simulink model "SimuOrbital"  (R2020b)
settings: Solver=VariableStepAuto  StartTime=0.0  StopTime=20000  RelTol=1e-3
model workspace (MAT data in the model file):
  Ang0 = [0; 0; 0]
  VelAng0 = [0; 0; 0]
  altura = 3.5
  delta = 0.05
  mu = 0.01
  r = 2.25
  radio = 2.25
libraries: sharedutil x11, aerolibutil x4, simulink_extras x3, sharedtransform x3, aerolibbdyn x2, vrlib x1, simulink x1
settings Model: Creator=Sergio  LastModifiedBy=Sergio
settings SolverCC: ZeroCrossAlgorithm=Adaptive

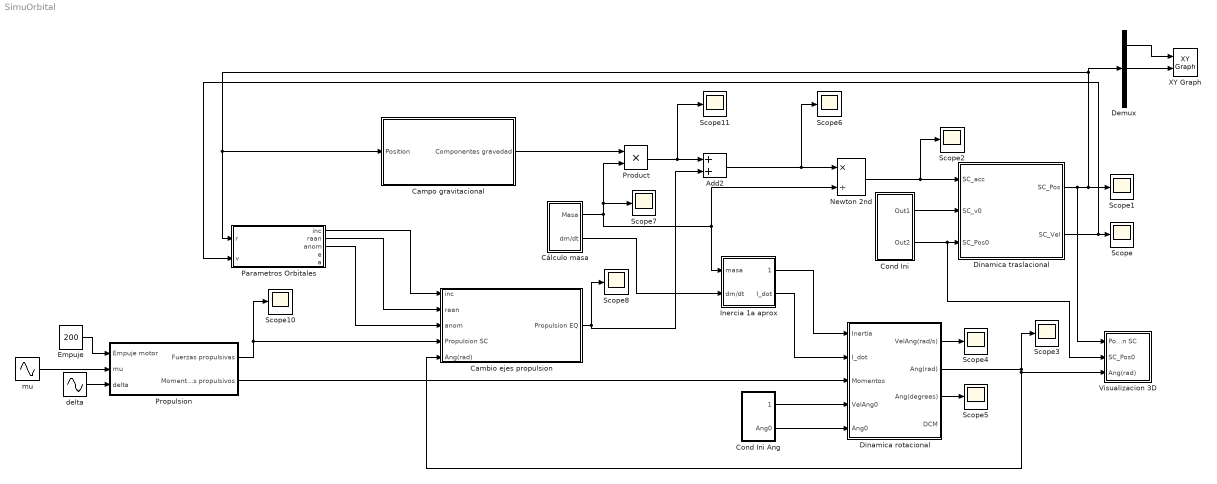
== system SimuOrbital ==
  Add2 : Sum
  Cambio ejes propulsion : Subsystem
  Campo gravitacional : Subsystem
  Cond Ini : Subsystem  mask{v0=[-1636,0,0], Pos0=[0,1837100,0]}
  Cond Ini Ang : Subsystem  mask{VelAng0=[0,0,0], Ang0=[0,0,0]}
  Cálculo masa : Subsystem
  Demux : Demux  Outputs=3
  Dinamica rotacional : Subsystem
  Dinamica traslacional : Subsystem
  Empuje : Constant  Value=200
  Inercia 1a aprox : Subsystem
  Newton 2nd : Product  Inputs=*/
  Parametros Orbitales : Subsystem
  Product : Product
  Propulsion : Subsystem
  Scope{,1..8,10..11} (11 alike) : Scope
  Visualizacion 3D : Subsystem
  XY Graph : simulink/Sinks/XY Graph  xmin=-2500000  xmax=2500000  ymin=-2500000  ymax=2500000  st=-1
  delta : Sin  Amplitude=0.01  Frequency=0.001  SampleTime=0
  mu : Sin  Amplitude=0.05  Frequency=0.001  SampleTime=0
  wires:
  Cond Ini/1(Out1) -> Dinamica traslacional/2(SC_v0)
  Cond Ini/2(Out2) -> Visualizacion 3D/2(SC_Pos0), Dinamica traslacional/3(SC_Pos0)
  Newton 2nd/1 -> Scope2/1, Dinamica traslacional/1(SC_acc)
  Dinamica traslacional/2(SC_Vel) -> Parametros Orbitales/2(v), Scope/1
  Inercia 1a aprox/1(Inertia) -> Dinamica rotacional/1(Inertia)
  Dinamica rotacional/1(VelAng(rad/s)) -> Scope4/1
  Cond Ini Ang/1(VelAng0) -> Dinamica rotacional/4(VelAng0)
  Cond Ini Ang/2(Ang0) -> Dinamica rotacional/5(Ang0)
  Dinamica rotacional/3(Ang(degrees)) -> Scope5/1
  Empuje/1 -> Propulsion/1(Empuje motor)
  Campo gravitacional/1(Componentes gravedad) -> Product/1
  Add2/1 -> Scope6/1, Newton 2nd/1
  Dinamica traslacional/1(SC_Pos) -> Visualizacion 3D/1(Posicion SC), Demux/1, Campo gravitacional/1(Position), Parametros Orbitales/1(r), Scope1/1
  Demux/1 -> XY Graph/1
  Demux/2 -> XY Graph/2
  Cambio ejes propulsion/1(Propulsion EQ) -> Add2/2, Scope8/1
  Parametros Orbitales/2(raan) -> Cambio ejes propulsion/2(raan)
  Parametros Orbitales/1(inc) -> Cambio ejes propulsion/1(inc)
  Parametros Orbitales/3(anom) -> Cambio ejes propulsion/3(anom)
  Dinamica rotacional/2(Ang(rad)) -> Cambio ejes propulsion/5(Ang(rad)), Visualizacion 3D/3(Ang(rad)), Scope3/1
  Propulsion/1(Fuerzas propulsivas) -> Scope10/1, Cambio ejes propulsion/4(Propulsion SC)
  Inercia 1a aprox/2(I_dot) -> Dinamica rotacional/2(I_dot)
  Cálculo masa/1(Masa) -> Inercia 1a aprox/1(masa), Newton 2nd/2, Scope7/1, Product/2
  Cálculo masa/2(dm/dt) -> Inercia 1a aprox/2(dm/dt)
  Product/1 -> Scope11/1, Add2/1
  Propulsion/2(Momentos propulsivos) -> Dinamica rotacional/3(Momentos)
  mu/1 -> Propulsion/2(mu)
  delta/1 -> Propulsion/3(delta)

== system SimuOrbital/Cambio ejes propulsion ==
  inc : Inport
  raan : Inport  Port=2
  anom : Inport  Port=3
  Propulsion SC : Inport  Port=4
  Ang(rad) : Inport  Port=5
  MATLAB Function : MATLAB Function  Commented=on  TreatAsAtomicUnit=on
  MatrixMultiply : Product  Inputs=3  Multiplication=Matrix(*)
  Product2 : Product  Multiplication=Matrix(*)
  Subsystem : Subsystem
  Subsystem1 : Subsystem
  Subsystem2 : Subsystem
  Propulsion EQ : Outport
  wires:
  inc/1 -> Subsystem/1(inc)
  raan/1 -> Subsystem/2(raan)
  anom/1 -> Subsystem1/1(anom)
  Ang(rad)/1 -> Subsystem2/1(ang)
  Subsystem/1(Ropeq) -> MatrixMultiply/1
  Subsystem1/1(Rloop) -> MatrixMultiply/2
  MatrixMultiply/1 -> Product2/1
  Product2/1 -> Propulsion EQ/1
  Subsystem2/1(Ralo) -> MatrixMultiply/3
  Propulsion SC/1 -> Product2/2

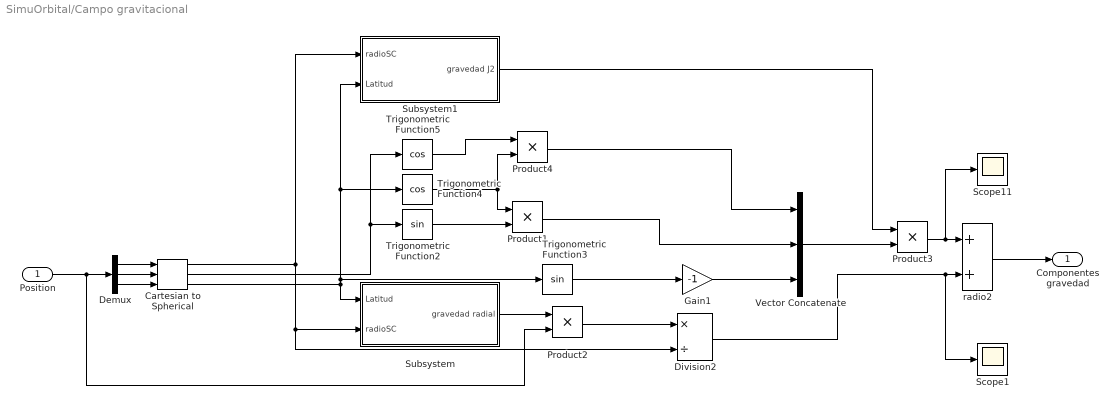
== system SimuOrbital/Campo gravitacional ==
  Position : Inport
  Cartesian to Spherical : simulink_extras/Transformations/Cartesian to Spherical
      settings: SourceProductBaseCode=SL
  Demux : Demux  Outputs=3
  Division2 : Product  Inputs=*/
  Gain1 : Gain  Gain=-1
  Product{1..4} (4 alike) : Product
  Scope1 : Scope
  Scope11 : Scope
  Subsystem : Subsystem
  Subsystem1 : Subsystem
  Trigonometric Function2 : Trigonometry
  Trigonometric Function3 : Trigonometry
  Trigonometric Function4 : Trigonometry  Operator=cos
  Trigonometric Function5 : Trigonometry  Operator=cos
  Vector Concatenate : Concatenate  NumInputs=3
  radio2 : Sum
  Componentes gravedad : Outport
  wires:
  Cartesian to Spherical/3 -> Subsystem/1(Latitud), Subsystem1/2(Latitud), Trigonometric Function4/1, Trigonometric Function3/1
  Position/1 -> Product2/2, Demux/1
  Cartesian to Spherical/1 -> Subsystem/2(radioSC), Division2/2, Subsystem1/1(radioSC)
  Product2/1 -> Division2/1
  Demux/2 -> Cartesian to Spherical/2
  Demux/1 -> Cartesian to Spherical/1
  Demux/3 -> Cartesian to Spherical/3
  Subsystem/1(gravedad radial) -> Product2/1
  Division2/1 -> Scope1/1, radio2/2
  radio2/1 -> Componentes gravedad/1
  Product3/1 -> Scope11/1, radio2/1
  Subsystem1/1(gravedad J2) -> Product3/1
  Trigonometric Function4/1 -> Product4/2, Product1/1
  Trigonometric Function2/1 -> Product1/2
  Cartesian to Spherical/2 -> Trigonometric Function5/1, Trigonometric Function2/1
  Trigonometric Function5/1 -> Product4/1
  Product4/1 -> Vector Concatenate/1
  Product1/1 -> Vector Concatenate/2
  Gain1/1 -> Vector Concatenate/3
  Trigonometric Function3/1 -> Gain1/1
  Vector Concatenate/1 -> Product3/2

== system SimuOrbital/Cond Ini ==
  SC_Pos0 : Constant  Value=Pos0  VectorParams1D=off
  SC_v0 : Constant  Value=v0  VectorParams1D=off
  Out1 : Outport
  Out2 : Outport  Port=2
  wires:
  SC_Pos0/1 -> Out2/1
  SC_v0/1 -> Out1/1

== system SimuOrbital/Cond Ini Ang ==
  CIAng : Constant  Value=Ang0  VectorParams1D=off
  CIVelAng : Constant  Value=VelAng0  VectorParams1D=off
  VelAng0 : Outport
  Ang0 : Outport  Port=2
  wires:
  CIVelAng/1 -> VelAng0/1
  CIAng/1 -> Ang0/1

== system SimuOrbital/Cálculo masa ==
  Add : Sum  Inputs=+-
  Constant : Constant
  Integrator : Integrator
  Masa inicial : Constant  Value=5000
  Masa seca : Constant  Value=2530
  Product : Product
  Switch : Switch  Criteria=u2 > Threshold  Threshold=2530
  dm/dt (kg/s) : Constant  Value=0
  Masa : Outport
  dm/dt : Outport  Port=2
  wires:
  dm/dt (kg/s)/1 -> Product/2, dm/dt/1
  Masa seca/1 -> Switch/3
  Switch/1 -> Masa/1
  Constant/1 -> Integrator/1
  Integrator/1 -> Product/1
  Product/1 -> Add/2
  Masa inicial/1 -> Add/1
  Add/1 -> Switch/2, Switch/1

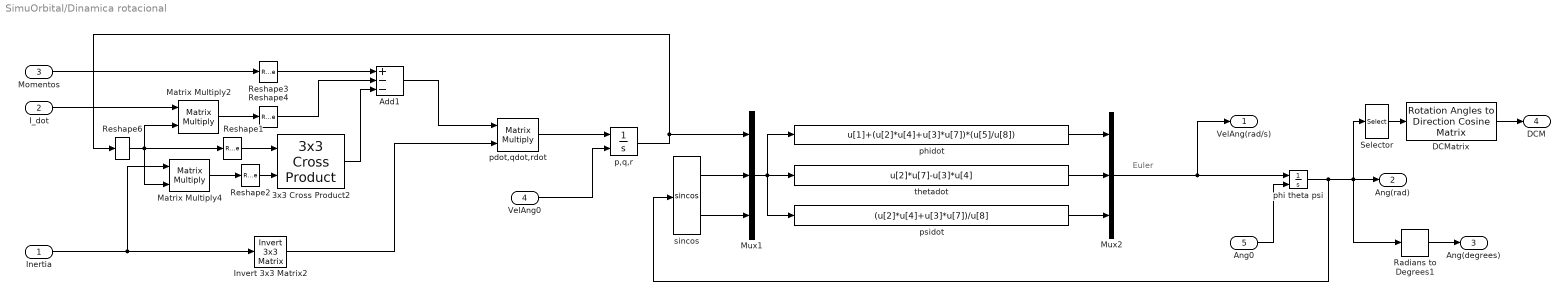
== system SimuOrbital/Dinamica rotacional ==
  note: Euler
  Inertia : Inport
  I_dot : Inport  Port=2
  Momentos : Inport  Port=3
  VelAng0 : Inport  Port=4
  Ang0 : Inport  Port=5
  3x3 Cross Product2 : sharedutil/3x3 Cross Product  aMode=aMode
      settings: SourceProductBaseCode=AE,PW,MT,UV,VE,VP
  Add1 : Sum  Inputs=+--
  DCMatrix : sharedtransform/Rotation Angles to Direction Cosine Matrix  rotationOrder=ZYX  aMode=aMode
      settings: SourceProductBaseCode=AE,PW,MT,UV,VE,VP
  Invert 3x3 Matrix2 : aerolibutil/Invert  3x3 Matrix
  Matrix Multiply2 : Product  Multiplication=Matrix(*)
  Matrix Multiply4 : Product  Multiplication=Matrix(*)
  Mux1 : Mux  Inputs=[3 3 3]
  Mux2 : Mux  Inputs=3
  Radians to Degrees1 : simulink_extras/Transformations/Radians to Degrees
  Reshape{1..4} (4 alike) : Reshape  OutputDimensionality=Row vector (2-D)
  Reshape6 : Reshape  OutputDimensionality=Column vector (2-D)
  Selector : Selector  InputPortWidth=3  IndexOptions=Index vector (dialog)  Indices=[3 2 1]  OutputSizes=1
  p,q,r : Integrator  InitialConditionSource=external
  pdot,qdot,rdot : Product  Multiplication=Matrix(*)
  phi theta psi : Integrator  InitialConditionSource=external  WrapState=on
  phidot : Fcn  Expr=u[1]+(u[2]*u[4]+u[3]*u[7])*(u[5]/u[8])
  psidot : Fcn  Expr=(u[2]*u[4]+u[3]*u[7])/u[8]
  sincos : Trigonometry  Operator=sincos
  thetadot : Fcn  Expr=u[2]*u[7]-u[3]*u[4]
  VelAng(rad/s) : Outport
  Ang(rad) : Outport  Port=2
  Ang(degrees) : Outport  Port=3
  DCM : Outport  Port=4
  wires:
  Invert 3x3 Matrix2/1 -> pdot,qdot,rdot/2
  Inertia/1 -> Matrix Multiply4/1, Invert 3x3 Matrix2/1
  Add1/1 -> pdot,qdot,rdot/1
  pdot,qdot,rdot/1 -> p,q,r/1
  I_dot/1 -> Matrix Multiply2/1
  3x3 Cross Product2/1 -> Add1/3
  Mux1/1 -> thetadot/1, phidot/1, psidot/1
  sincos/2 -> Mux1/3
  sincos/1 -> Mux1/2
  thetadot/1 -> Mux2/2
  phidot/1 -> Mux2/1
  psidot/1 -> Mux2/3
  Radians to Degrees1/1 -> Ang(degrees)/1
  Ang0/1 -> phi theta psi/2
  Mux2/1 -> phi theta psi/1, VelAng(rad/s)/1
  p,q,r/1 -> Reshape6/1, Mux1/1
  Reshape1/1 -> 3x3 Cross Product2/1
  Matrix Multiply4/1 -> Reshape2/1
  Reshape2/1 -> 3x3 Cross Product2/2
  Reshape3/1 -> Add1/1
  Momentos/1 -> Reshape3/1
  Matrix Multiply2/1 -> Reshape4/1
  Reshape4/1 -> Add1/2
  VelAng0/1 -> p,q,r/2
  Reshape6/1 -> Matrix Multiply2/2, Matrix Multiply4/2, Reshape1/1
  phi theta psi/1 -> Radians to Degrees1/1, Selector/1, Ang(rad)/1, sincos/1
  Selector/1 -> DCMatrix/1
  DCMatrix/1 -> DCM/1

== system SimuOrbital/Dinamica traslacional ==
  SC_acc : Inport
  SC_v0 : Inport  Port=2
  SC_Pos0 : Inport  Port=3
  Add : Sum
  Add1 : Sum
  Integrator : Integrator
  Integrator1 : Integrator
  SC_Pos : Outport
  SC_Vel : Outport  Port=2
  wires:
  Add/1 -> SC_Vel/1, Integrator1/1
  Add1/1 -> SC_Pos/1
  SC_Pos0/1 -> Add1/2
  SC_acc/1 -> Integrator/1
  SC_v0/1 -> Add/2
  Integrator/1 -> Add/1
  Integrator1/1 -> Add1/1

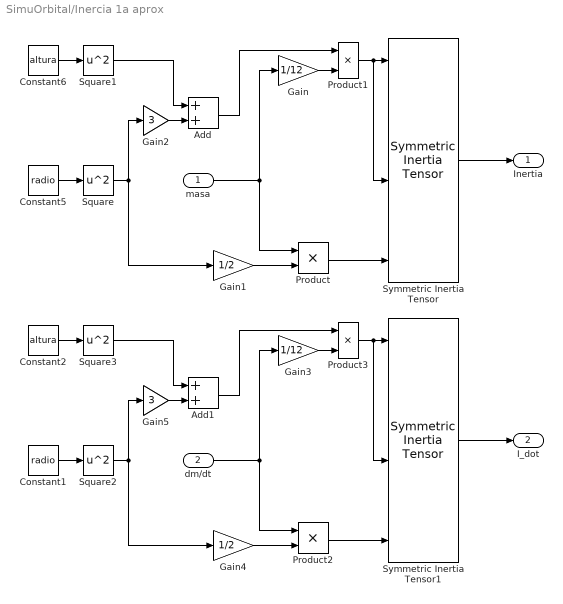
== system SimuOrbital/Inercia 1a aprox ==
  masa : Inport
  dm/dt : Inport  Port=2
  Add : Sum
  Add1 : Sum
  Constant1 : Constant  Value=radio
  Constant2 : Constant  Value=altura
  Constant5 : Constant  Value=radio
  Constant6 : Constant  Value=altura
  Gain : Gain  Gain=1/12
  Gain1 : Gain  Gain=1/2
  Gain2 : Gain  Gain=3
  Gain3 : Gain  Gain=1/12
  Gain4 : Gain  Gain=1/2
  Gain5 : Gain  Gain=3
  Product{,1..3} (4 alike) : Product
  Square{,1..3} (4 alike) : Math  Operator=square  SaturateOnIntegerOverflow=on
  Symmetric Inertia Tensor : aerolibbdyn/Symmetric Inertia Tensor
      settings: SourceProductBaseCode=AE
  Symmetric Inertia Tensor1 : aerolibbdyn/Symmetric Inertia Tensor
      settings: SourceProductBaseCode=AE
  Inertia : Outport
  I_dot : Outport  Port=2
  wires:
  Gain2/1 -> Add/2
  Square1/1 -> Add/1
  Product/1 -> Symmetric Inertia Tensor/6
  masa/1 -> Gain/1, Product/1
  Gain/1 -> Product1/2
  Symmetric Inertia Tensor/1 -> Inertia/1
  Square/1 -> Gain2/1, Gain1/1
  Add/1 -> Product1/1
  Product1/1 -> Symmetric Inertia Tensor/4, Symmetric Inertia Tensor/1
  Gain1/1 -> Product/2
  Constant5/1 -> Square/1
  Constant6/1 -> Square1/1
  Constant1/1 -> Square2/1
  Square2/1 -> Gain5/1, Gain4/1
  Constant2/1 -> Square3/1
  Square3/1 -> Add1/1
  Product3/1 -> Symmetric Inertia Tensor1/4, Symmetric Inertia Tensor1/1
  Gain5/1 -> Add1/2
  Gain3/1 -> Product3/2
  Gain4/1 -> Product2/2
  Product2/1 -> Symmetric Inertia Tensor1/6
  Add1/1 -> Product3/1
  dm/dt/1 -> Gain3/1, Product2/1
  Symmetric Inertia Tensor1/1 -> I_dot/1

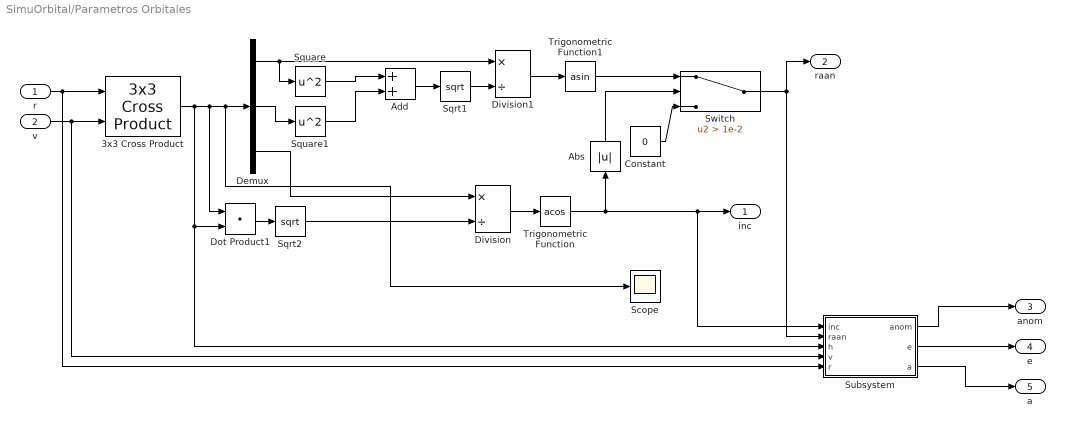
== system SimuOrbital/Parametros Orbitales ==
  r : Inport
  v : Inport  Port=2
  3x3 Cross Product : sharedutil/3x3 Cross Product  aMode=aMode
      settings: SourceProductBaseCode=AE,PW,MT,UV,VE,VP
  Abs : Abs
  Add : Sum
  Constant : Constant  Value=0
  Demux : Demux  Outputs=3
  Division : Product  Inputs=*/
  Division1 : Product  Inputs=*/
  Dot Product1 : DotProduct  InputSameDT=on  OutDataTypeStr=Inherit: Inherit via internal rule
  Scope : Scope
  Sqrt1 : Sqrt  SaturateOnIntegerOverflow=on
  Sqrt2 : Sqrt  SaturateOnIntegerOverflow=on
  Square : Math  Operator=square  SaturateOnIntegerOverflow=on
  Square1 : Math  Operator=square  SaturateOnIntegerOverflow=on
  Subsystem : Subsystem
  Switch : Switch  Criteria=u2 > Threshold  Threshold=1e-2
  Trigonometric Function : Trigonometry  Operator=acos
  Trigonometric Function1 : Trigonometry  Operator=asin
  inc : Outport
  raan : Outport  Port=2
  anom : Outport  Port=3
  e : Outport  Port=4
  a : Outport  Port=5
  wires:
  r/1 -> Subsystem/5(r), 3x3 Cross Product/1
  Trigonometric Function/1 -> Abs/1, Subsystem/1(inc), inc/1
  Division/1 -> Trigonometric Function/1
  Demux/3 -> Division/1
  Sqrt2/1 -> Division/2
  Switch/1 -> Subsystem/2(raan), raan/1
  Dot Product1/1 -> Sqrt2/1
  v/1 -> Subsystem/4(v), 3x3 Cross Product/2
  Constant/1 -> Switch/3
  Trigonometric Function1/1 -> Switch/1
  Abs/1 -> Switch/2
  Division1/1 -> Trigonometric Function1/1
  Demux/1 -> Square/1, Division1/1
  Sqrt1/1 -> Division1/2
  Add/1 -> Sqrt1/1
  Demux/2 -> Square1/1
  Square1/1 -> Add/2
  Square/1 -> Add/1
  Subsystem/2(e) -> e/1
  Subsystem/1(anom) -> anom/1
  Subsystem/3(a) -> a/1
  3x3 Cross Product/1 -> Subsystem/3(h), Dot Product1/2, Dot Product1/1, Scope/1, Demux/1

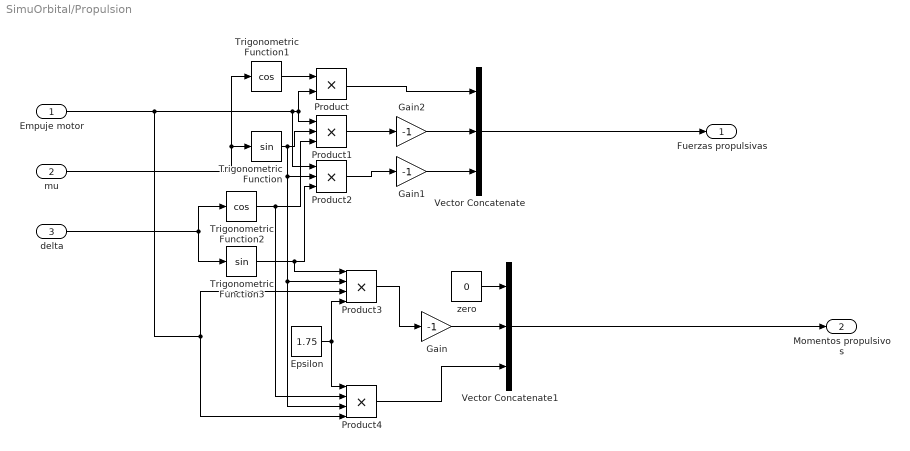
== system SimuOrbital/Propulsion ==
  Empuje motor : Inport
  mu : Inport  Port=2
  delta : Inport  Port=3
  Epsilon : Constant  Value=1.75
  Gain : Gain  Gain=-1
  Gain1 : Gain  Gain=-1
  Gain2 : Gain  Gain=-1
  Product : Product
  Product1 : Product  Inputs=3
  Product2 : Product  Inputs=3
  Product3 : Product  Inputs=4
  Product4 : Product  Inputs=4
  Trigonometric Function : Trigonometry
  Trigonometric Function1 : Trigonometry  Operator=cos
  Trigonometric Function2 : Trigonometry  Operator=cos
  Trigonometric Function3 : Trigonometry
  Vector Concatenate : Concatenate  NumInputs=3
  Vector Concatenate1 : Concatenate  NumInputs=3
  zero : Constant  Value=0
  Fuerzas propulsivas : Outport
  Momentos propulsivos : Outport  Port=2
  wires:
  Product4/1 -> Vector Concatenate1/3
  zero/1 -> Vector Concatenate1/1
  Trigonometric Function1/1 -> Product/1
  Vector Concatenate1/1 -> Momentos propulsivos/1
  delta/1 -> Trigonometric Function2/1, Trigonometric Function3/1
  Trigonometric Function/1 -> Product4/3, Product3/2, Product2/2, Product1/2
  Empuje motor/1 -> Product4/4, Product3/3, Product2/1, Product/2, Product1/1
  Trigonometric Function3/1 -> Product3/1, Product2/3
  mu/1 -> Trigonometric Function/1, Trigonometric Function1/1
  Trigonometric Function2/1 -> Product4/2, Product1/3
  Epsilon/1 -> Product3/4, Product4/1
  Product/1 -> Vector Concatenate/1
  Vector Concatenate/1 -> Fuerzas propulsivas/1
  Gain1/1 -> Vector Concatenate/3
  Gain2/1 -> Vector Concatenate/2
  Product1/1 -> Gain2/1
  Product2/1 -> Gain1/1
  Gain/1 -> Vector Concatenate1/2
  Product3/1 -> Gain/1

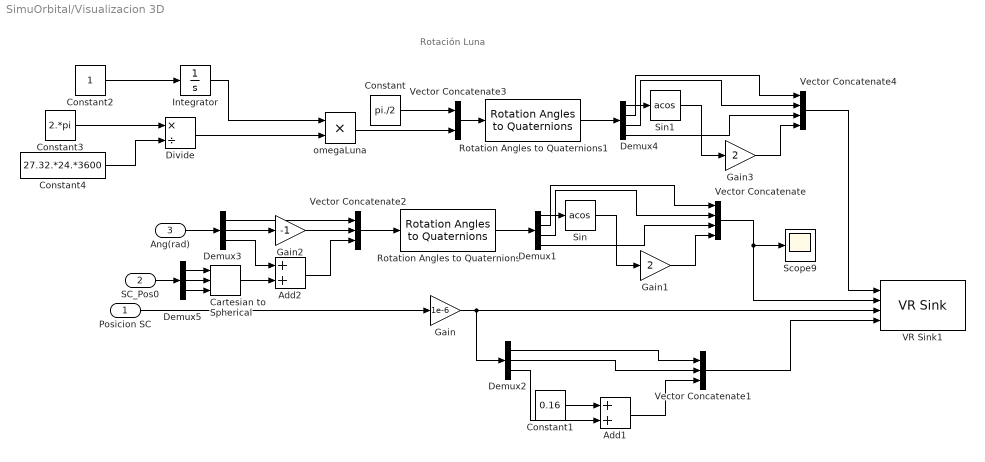
== system SimuOrbital/Visualizacion 3D ==
  note: Rotación Luna
  Posicion SC : Inport
  SC_Pos0 : Inport  Port=2
  Ang(rad) : Inport  Port=3
  Add1 : Sum
  Add2 : Sum
  Cartesian to Spherical : simulink_extras/Transformations/Cartesian to Spherical
      settings: SourceProductBaseCode=SL
  Constant : Constant  Value=pi./2
  Constant1 : Constant  Value=0.16
  Constant2 : Constant
  Constant3 : Constant  Value=2.*pi
  Constant4 : Constant  Value=27.32.*24.*3600
  Demux1 : Demux
  Demux2 : Demux  Outputs=3
  Demux3 : Demux  Outputs=3
  Demux4 : Demux
  Demux5 : Demux  Outputs=3
  Divide : Product  Inputs=*/
  Gain : Gain  Gain=1e-6
  Gain1 : Gain  Gain=2
  Gain2 : Gain  Gain=-1
  Gain3 : Gain  Gain=2
  Integrator : Integrator
  Rotation Angles to Quaternions : sharedtransform/Rotation Angles to Quaternions  rotationOrder=ZYZ  aMode=aMode
      settings: SourceProductBaseCode=AE,PW,MT,UV,VE,VP
  Rotation Angles to Quaternions1 : sharedtransform/Rotation Angles to Quaternions  rotationOrder=XYZ  aMode=aMode
      settings: SourceProductBaseCode=AE,PW,MT,UV,VE,VP
  Scope9 : Scope
  Sin : Trigonometry  Operator=acos
  Sin1 : Trigonometry  Operator=acos
  VR Sink1 : vrlib/VR Sink  InstantiateOnLoad=on  SampleTime=0.1  ViewEnable=on  RemoteChange=off  RemoteView=off  FieldsWritten=MOON.rotation.4.1.1.double#SC.rotation.4.1.1.double#SC.translation.3.1.1.double#Orbita_0001.position.3.1.1.double  WorldFileName=orbita.x3d  AutoView=off  VideoDimensions=[]  AllowVariableSize=off
  Vector Concatenate : Concatenate  NumInputs=4
  Vector Concatenate1 : Concatenate  NumInputs=3
  Vector Concatenate2 : Concatenate  NumInputs=3
  Vector Concatenate3 : Concatenate  NumInputs=3
  Vector Concatenate4 : Concatenate  NumInputs=4
  omegaLuna : Product
  wires:
  Constant1/1 -> Add1/1
  Demux2/2 -> Vector Concatenate1/2
  Demux1/3 -> Vector Concatenate/2
  Vector Concatenate1/1 -> VR Sink1/4
  Demux1/1 -> Sin/1
  Demux2/3 -> Add1/2
  Add1/1 -> Vector Concatenate1/3
  Gain/1 -> VR Sink1/3, Demux2/1
  Gain1/1 -> Vector Concatenate/4
  Demux1/4 -> Vector Concatenate/3
  Vector Concatenate/1 -> VR Sink1/2, Scope9/1
  Sin/1 -> Gain1/1
  Demux2/1 -> Vector Concatenate1/1
  Rotation Angles to Quaternions/1 -> Demux1/1
  Demux1/2 -> Vector Concatenate/1
  Posicion SC/1 -> Gain/1
  Ang(rad)/1 -> Demux3/1
  Vector Concatenate2/1 -> Rotation Angles to Quaternions/1
  Demux3/1 -> Vector Concatenate2/1
  Gain2/1 -> Vector Concatenate2/2
  Demux3/2 -> Gain2/1
  Vector Concatenate3/1 -> Rotation Angles to Quaternions1/1
  Rotation Angles to Quaternions1/1 -> Demux4/1
  Sin1/1 -> Gain3/1
  Demux4/2 -> Vector Concatenate4/1
  Gain3/1 -> Vector Concatenate4/4
  Demux4/3 -> Vector Concatenate4/2
  Demux4/4 -> Vector Concatenate4/3
  Demux4/1 -> Sin1/1
  Constant/1 -> Vector Concatenate3/1
  omegaLuna/1 -> Vector Concatenate3/3
  Constant2/1 -> Integrator/1
  Integrator/1 -> omegaLuna/1
  Divide/1 -> omegaLuna/2
  Constant3/1 -> Divide/1
  Constant4/1 -> Divide/2
  Vector Concatenate4/1 -> VR Sink1/1
  Demux3/3 -> Add2/1
  Add2/1 -> Vector Concatenate2/3
  Demux5/1 -> Cartesian to Spherical/1
  Demux5/2 -> Cartesian to Spherical/2
  Demux5/3 -> Cartesian to Spherical/3
  Cartesian to Spherical/2 -> Add2/2
  SC_Pos0/1 -> Demux5/1

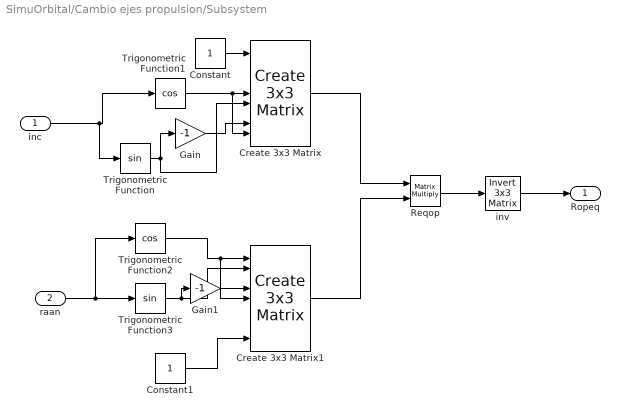
== system SimuOrbital/Cambio ejes propulsion/Subsystem ==
  inc : Inport
  raan : Inport  Port=2
  Constant : Constant
  Constant1 : Constant
  Create 3x3 Matrix : sharedutil/Create 3x3 Matrix  aMode=aMode
      settings: SourceProductBaseCode=AE,PW,MT,UV,VE,VP
  Create 3x3 Matrix1 : sharedutil/Create 3x3 Matrix  aMode=aMode
      settings: SourceProductBaseCode=AE,PW,MT,UV,VE,VP
  Gain : Gain  Gain=-1
  Gain1 : Gain  Gain=-1
  Reqop : Product  Multiplication=Matrix(*)
  Trigonometric Function : Trigonometry
  Trigonometric Function1 : Trigonometry  Operator=cos
  Trigonometric Function2 : Trigonometry  Operator=cos
  Trigonometric Function3 : Trigonometry
  inv : aerolibutil/Invert  3x3 Matrix
  Ropeq : Outport
  wires:
  Constant/1 -> Create 3x3 Matrix/1
  Trigonometric Function1/1 -> Create 3x3 Matrix/9, Create 3x3 Matrix/5
  inc/1 -> Trigonometric Function/1, Trigonometric Function1/1
  Trigonometric Function/1 -> Gain/1, Create 3x3 Matrix/6
  Constant1/1 -> Create 3x3 Matrix1/9
  Trigonometric Function2/1 -> Create 3x3 Matrix1/5, Create 3x3 Matrix1/1
  Trigonometric Function3/1 -> Gain1/1, Create 3x3 Matrix1/2
  Gain1/1 -> Create 3x3 Matrix1/4
  raan/1 -> Trigonometric Function2/1, Trigonometric Function3/1
  Create 3x3 Matrix/1 -> Reqop/1
  Create 3x3 Matrix1/1 -> Reqop/2
  Reqop/1 -> inv/1
  inv/1 -> Ropeq/1
  Gain/1 -> Create 3x3 Matrix/8

== system SimuOrbital/Cambio ejes propulsion/Subsystem1 ==
  anom : Inport
  Constant1 : Constant
  Constant2 : Constant
  Constant3 : Constant
  Create 3x3 Matrix1 : sharedutil/Create 3x3 Matrix  aMode=aMode
      settings: SourceProductBaseCode=AE,PW,MT,UV,VE,VP
  Create 3x3 Matrix2 : sharedutil/Create 3x3 Matrix  aMode=aMode
      settings: SourceProductBaseCode=AE,PW,MT,UV,VE,VP
  Create 3x3 Matrix3 : sharedutil/Create 3x3 Matrix  aMode=aMode
      settings: SourceProductBaseCode=AE,PW,MT,UV,VE,VP
  Gain1 : Gain  Gain=-1
  Gain2 : Gain  Gain=-1
  Gain3 : Gain  Gain=-1
  Roplo : Product  Inputs=3  Multiplication=Matrix(*)
  Trigonometric Function2 : Trigonometry  Operator=cos
  Trigonometric Function3 : Trigonometry
  inv : aerolibutil/Invert  3x3 Matrix
  Rloop : Outport
  wires:
  anom/1 -> Trigonometric Function2/1, Trigonometric Function3/1
  Constant3/1 -> Create 3x3 Matrix3/9
  Gain3/1 -> Create 3x3 Matrix3/4
  Trigonometric Function3/1 -> Gain3/1, Create 3x3 Matrix3/2
  Trigonometric Function2/1 -> Create 3x3 Matrix3/5, Create 3x3 Matrix3/1
  Create 3x3 Matrix2/1 -> Roplo/2
  Create 3x3 Matrix3/1 -> Roplo/3
  Create 3x3 Matrix1/1 -> Roplo/1
  inv/1 -> Rloop/1
  Roplo/1 -> inv/1
  Constant2/1 -> Create 3x3 Matrix2/8, Gain2/1, Create 3x3 Matrix2/1
  Gain2/1 -> Create 3x3 Matrix2/6
  Gain1/1 -> Create 3x3 Matrix1/7
  Constant1/1 -> Create 3x3 Matrix1/3, Create 3x3 Matrix1/5, Gain1/1

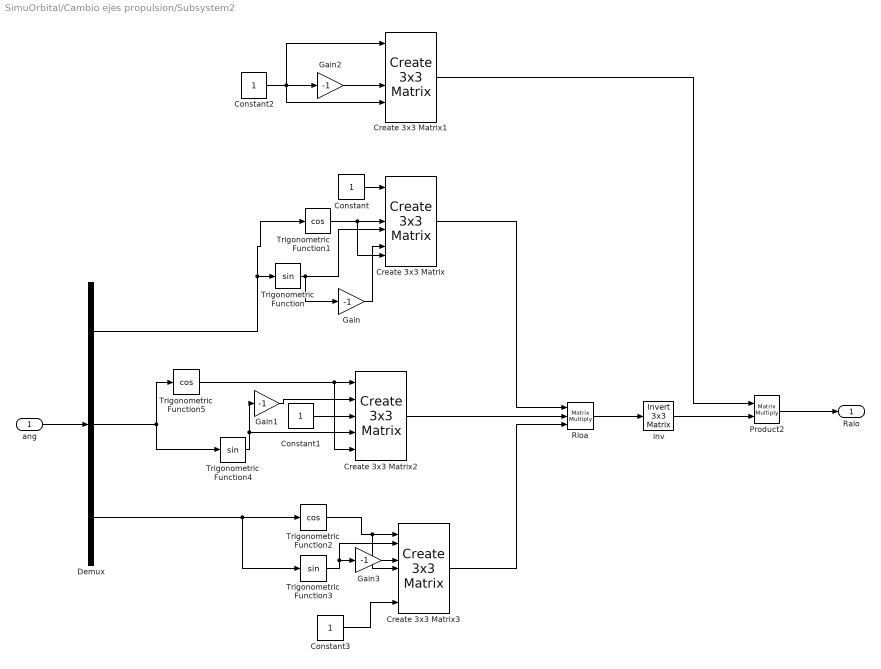
== system SimuOrbital/Cambio ejes propulsion/Subsystem2 ==
  ang : Inport
  Constant{,1..3} (4 alike) : Constant
  Create 3x3 Matrix{,1..3} (4 alike) : sharedutil/Create 3x3 Matrix  aMode=aMode
      settings: SourceProductBaseCode=AE,PW,MT,UV,VE,VP
  Demux : Demux  Outputs=3
  Gain{,1..3} (4 alike) : Gain  Gain=-1
  Product2 : Product  Multiplication=Matrix(*)
  Rloa : Product  Inputs=3  Multiplication=Matrix(*)
  Trigonometric Function : Trigonometry
  Trigonometric Function1 : Trigonometry  Operator=cos
  Trigonometric Function2 : Trigonometry  Operator=cos
  Trigonometric Function3 : Trigonometry
  Trigonometric Function4 : Trigonometry
  Trigonometric Function5 : Trigonometry  Operator=cos
  inv : aerolibutil/Invert  3x3 Matrix
  Ralo : Outport
  wires:
  Create 3x3 Matrix2/1 -> Rloa/2
  Constant3/1 -> Create 3x3 Matrix3/9
  Gain3/1 -> Create 3x3 Matrix3/4
  Trigonometric Function3/1 -> Gain3/1, Create 3x3 Matrix3/2
  Create 3x3 Matrix3/1 -> Rloa/3
  Trigonometric Function2/1 -> Create 3x3 Matrix3/5, Create 3x3 Matrix3/1
  ang/1 -> Demux/1
  Trigonometric Function/1 -> Create 3x3 Matrix/6, Gain/1
  Constant/1 -> Create 3x3 Matrix/1
  Trigonometric Function1/1 -> Create 3x3 Matrix/9, Create 3x3 Matrix/5
  Demux/1 -> Trigonometric Function1/1, Trigonometric Function/1
  Create 3x3 Matrix/1 -> Rloa/1
  Demux/3 -> Trigonometric Function3/1, Trigonometric Function2/1
  Constant1/1 -> Create 3x3 Matrix2/5
  Demux/2 -> Trigonometric Function4/1, Trigonometric Function5/1
  Trigonometric Function4/1 -> Create 3x3 Matrix2/7, Gain1/1
  Gain1/1 -> Create 3x3 Matrix2/3
  Trigonometric Function5/1 -> Create 3x3 Matrix2/9, Create 3x3 Matrix2/1
  Gain/1 -> Create 3x3 Matrix/8
  Constant2/1 -> Create 3x3 Matrix1/8, Create 3x3 Matrix1/1, Gain2/1
  Create 3x3 Matrix1/1 -> Product2/1
  Product2/1 -> Ralo/1
  inv/1 -> Product2/2
  Rloa/1 -> inv/1
  Gain2/1 -> Create 3x3 Matrix1/6

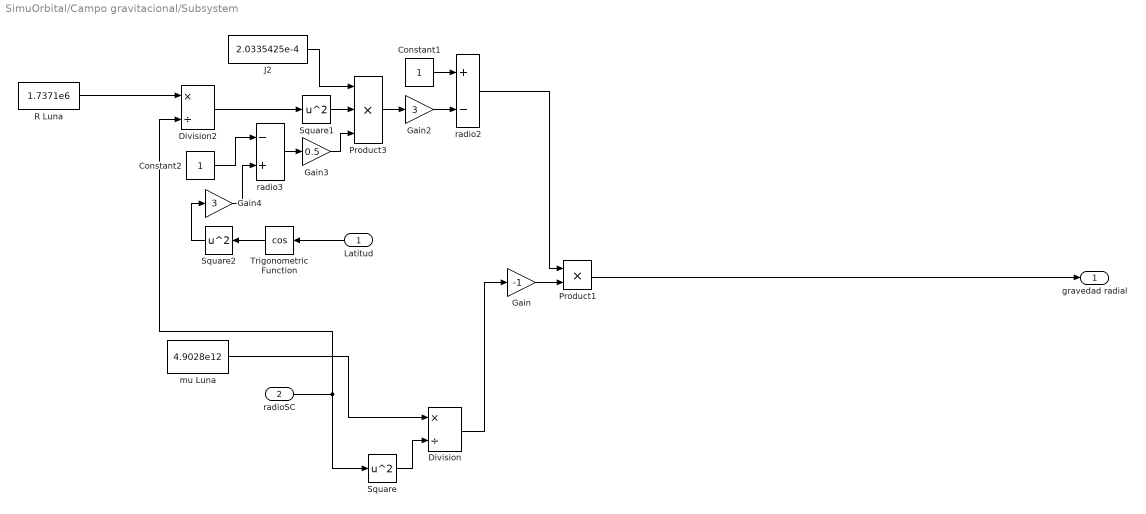
== system SimuOrbital/Campo gravitacional/Subsystem ==
  Latitud : Inport
  radioSC : Inport  Port=2
  Constant1 : Constant
  Constant2 : Constant
  Division : Product  Inputs=*/
  Division2 : Product  Inputs=*/
  Gain : Gain  Gain=-1
  Gain2 : Gain  Gain=3
  Gain3 : Gain  Gain=0.5
  Gain4 : Gain  Gain=3
  J2 : Constant  Value=2.0335425e-4
  Product1 : Product
  Product3 : Product  Inputs=3
  R Luna : Constant  Value=1.7371e6
  Square : Math  Operator=square  SaturateOnIntegerOverflow=on
  Square1 : Math  Operator=square  SaturateOnIntegerOverflow=on
  Square2 : Math  Operator=square  SaturateOnIntegerOverflow=on
  Trigonometric Function : Trigonometry  Operator=cos
  mu Luna : Constant  Value=4.9028e12
  radio2 : Sum  Inputs=+-
  radio3 : Sum  Inputs=-+
  gravedad radial : Outport
  wires:
  radio2/1 -> Product1/1
  R Luna/1 -> Division2/1
  mu Luna/1 -> Division/1
  Gain3/1 -> Product3/3
  radioSC/1 -> Square/1, Division2/2
  J2/1 -> Product3/1
  Division2/1 -> Square1/1
  Square1/1 -> Product3/2
  Division/1 -> Gain/1
  Constant1/1 -> radio2/1
  Latitud/1 -> Trigonometric Function/1
  Product3/1 -> Gain2/1
  Gain2/1 -> radio2/2
  Trigonometric Function/1 -> Square2/1
  Gain/1 -> Product1/2
  radio3/1 -> Gain3/1
  Square/1 -> Division/2
  Constant2/1 -> radio3/1
  Square2/1 -> Gain4/1
  Gain4/1 -> radio3/2
  Product1/1 -> gravedad radial/1

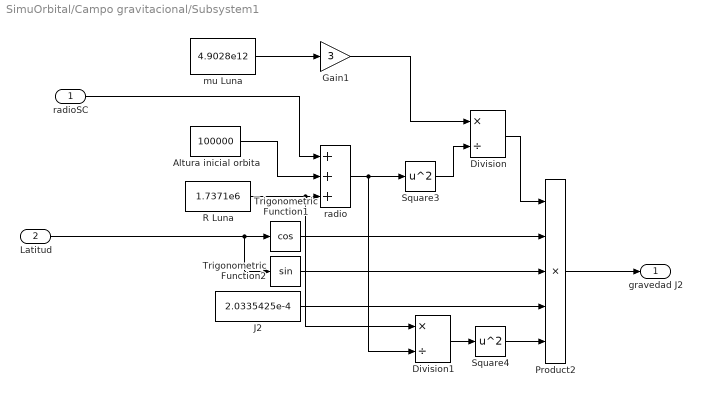
== system SimuOrbital/Campo gravitacional/Subsystem1 ==
  radioSC : Inport
  Latitud : Inport  Port=2
  Altura inicial orbita : Constant  Value=100000
  Division : Product  Inputs=*/
  Division1 : Product  Inputs=*/
  Gain1 : Gain  Gain=3
  J2 : Constant  Value=2.0335425e-4
  Product2 : Product  Inputs=5
  R Luna : Constant  Value=1.7371e6
  Square3 : Math  Operator=square  SaturateOnIntegerOverflow=on
  Square4 : Math  Operator=square  SaturateOnIntegerOverflow=on
  Trigonometric Function1 : Trigonometry  Operator=cos
  Trigonometric Function2 : Trigonometry
  mu Luna : Constant  Value=4.9028e12
  radio : Sum  Inputs=+++
  gravedad J2 : Outport
  wires:
  mu Luna/1 -> Gain1/1
  radioSC/1 -> radio/1
  R Luna/1 -> Division1/1, radio/3
  radio/1 -> Division1/2, Square3/1
  Division/1 -> Product2/1
  Square3/1 -> Division/2
  Altura inicial orbita/1 -> radio/2
  Gain1/1 -> Division/1
  Latitud/1 -> Trigonometric Function2/1, Trigonometric Function1/1
  Trigonometric Function1/1 -> Product2/2
  Trigonometric Function2/1 -> Product2/3
  J2/1 -> Product2/4
  Square4/1 -> Product2/5
  Division1/1 -> Square4/1
  Product2/1 -> gravedad J2/1

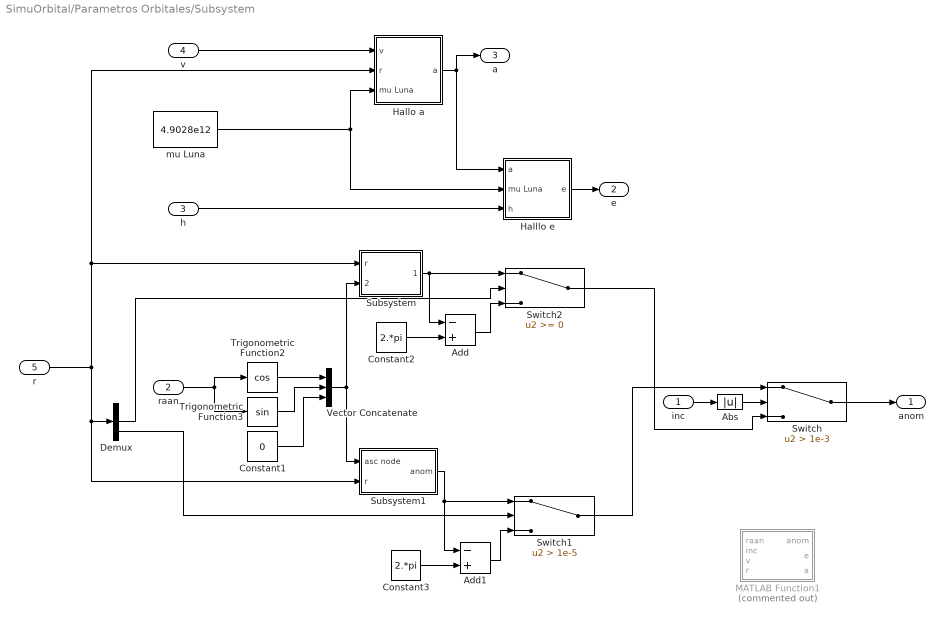
== system SimuOrbital/Parametros Orbitales/Subsystem ==
  inc : Inport
  raan : Inport  Port=2
  h : Inport  Port=3
  v : Inport  Port=4
  r : Inport  Port=5
  Abs : Abs
  Add : Sum  Inputs=-+
  Add1 : Sum  Inputs=-+
  Constant1 : Constant  Value=0
  Constant2 : Constant  Value=2.*pi
  Constant3 : Constant  Value=2.*pi
  Demux : Demux  Outputs=3
  Halllo e : Subsystem
  Hallo a : Subsystem
  MATLAB Function1 : MATLAB Function  Commented=on  TreatAsAtomicUnit=on
  Subsystem : Subsystem
  Subsystem1 : Subsystem
  Switch : Switch  Criteria=u2 > Threshold  Threshold=1e-3
  Switch1 : Switch  Criteria=u2 > Threshold  Threshold=1e-5
  Switch2 : Switch
  Trigonometric Function2 : Trigonometry  Operator=cos
  Trigonometric Function3 : Trigonometry
  Vector Concatenate : Concatenate  NumInputs=3
  mu Luna : Constant  Value=4.9028e12
  anom : Outport
  e : Outport  Port=2
  a : Outport  Port=3
  wires:
  Hallo a/1(a) -> Halllo e/1(a), a/1
  v/1 -> Hallo a/1(v)
  r/1 -> Hallo a/2(r), Subsystem/1(r), Subsystem1/2(r), Demux/1
  mu Luna/1 -> Hallo a/3(mu Luna), Halllo e/2(mu Luna)
  h/1 -> Halllo e/3(h)
  Halllo e/1(e) -> e/1
  inc/1 -> Abs/1
  Abs/1 -> Switch/2
  raan/1 -> Trigonometric Function3/1, Trigonometric Function2/1
  Trigonometric Function2/1 -> Vector Concatenate/1
  Trigonometric Function3/1 -> Vector Concatenate/2
  Constant1/1 -> Vector Concatenate/3
  Demux/3 -> Switch1/2
  Demux/2 -> Switch2/2
  Subsystem/1(anom) -> Add/1, Switch2/1
  Vector Concatenate/1 -> Subsystem1/1(asc node), Subsystem/2(asc node)
  Add/1 -> Switch2/3
  Constant2/1 -> Add/2
  Subsystem1/1(anom) -> Switch1/1, Add1/1
  Constant3/1 -> Add1/2
  Add1/1 -> Switch1/3
  Switch/1 -> anom/1
  Switch1/1 -> Switch/1
  Switch2/1 -> Switch/3

== system SimuOrbital/Parametros Orbitales/Subsystem/Halllo e ==
  a : Inport
  mu Luna : Inport  Port=2
  h : Inport  Port=3
  Constant1 : Constant
  Division4 : Product  Inputs=*/
  Dot Product3 : DotProduct  InputSameDT=on  OutDataTypeStr=Inherit: Inherit via internal rule
  Product1 : Product
  Sqrt1 : Sqrt  SaturateOnIntegerOverflow=on
  radio3 : Sum  Inputs=+-
  e : Outport
  wires:
  Dot Product3/1 -> Division4/1
  Constant1/1 -> radio3/1
  Product1/1 -> Division4/2
  Division4/1 -> radio3/2
  h/1 -> Dot Product3/2, Dot Product3/1
  radio3/1 -> Sqrt1/1
  Sqrt1/1 -> e/1
  mu Luna/1 -> Product1/2
  a/1 -> Product1/1

== system SimuOrbital/Parametros Orbitales/Subsystem/Hallo a ==
  v : Inport
  r : Inport  Port=2
  mu Luna : Inport  Port=3
  Division1 : Product  Inputs=*/
  Division3 : Product  Inputs=*/
  Dot Product1 : DotProduct  InputSameDT=on  OutDataTypeStr=Inherit: Inherit via internal rule
  Dot Product2 : DotProduct  InputSameDT=on  OutDataTypeStr=Inherit: Inherit via internal rule
  Gain2 : Gain  Gain=2
  Sqrt : Sqrt  SaturateOnIntegerOverflow=on
  radio2 : Sum  Inputs=+-
  a : Outport
  wires:
  v/1 -> Dot Product1/2, Dot Product1/1
  Dot Product1/1 -> radio2/2
  mu Luna/1 -> Gain2/1, Division1/1
  radio2/1 -> Division1/2
  r/1 -> Dot Product2/2, Dot Product2/1
  Gain2/1 -> Division3/1
  Division3/1 -> radio2/1
  Division1/1 -> a/1
  Dot Product2/1 -> Sqrt/1
  Sqrt/1 -> Division3/2

== system SimuOrbital/Parametros Orbitales/Subsystem/Subsystem ==
  r : Inport
  asc node : Inport  Port=2
  Divide : Product  Inputs=*/
  Dot Product : DotProduct  InputSameDT=on  OutDataTypeStr=Inherit: Inherit via internal rule
  Dot Product1 : DotProduct  InputSameDT=on  OutDataTypeStr=Inherit: Inherit via internal rule
  Sqrt : Sqrt  SaturateOnIntegerOverflow=on
  Trigonometric Function : Trigonometry  Operator=acos
  anom : Outport
  wires:
  Trigonometric Function/1 -> anom/1
  Divide/1 -> Trigonometric Function/1
  Sqrt/1 -> Divide/2
  Dot Product/1 -> Sqrt/1
  r/1 -> Dot Product/2, Dot Product1/2, Dot Product/1
  asc node/1 -> Dot Product1/1
  Dot Product1/1 -> Divide/1

== system SimuOrbital/Parametros Orbitales/Subsystem/Subsystem1 ==
  asc node : Inport
  r : Inport  Port=2
  Divide : Product  Inputs=*/
  Dot Product : DotProduct  InputSameDT=on  OutDataTypeStr=Inherit: Inherit via internal rule
  Dot Product1 : DotProduct  InputSameDT=on  OutDataTypeStr=Inherit: Inherit via internal rule
  Sqrt : Sqrt  SaturateOnIntegerOverflow=on
  Trigonometric Function : Trigonometry  Operator=acos
  anom : Outport
  wires:
  r/1 -> Dot Product1/2, Dot Product/1, Dot Product/2
  Divide/1 -> Trigonometric Function/1
  Dot Product/1 -> Sqrt/1
  Trigonometric Function/1 -> anom/1
  Sqrt/1 -> Divide/2
  asc node/1 -> Dot Product1/1
  Dot Product1/1 -> Divide/1

== matlab function SimuOrbital/Parametros Orbitales/Subsystem/MATLAB Function1 ==
  data: raan input; inc input; v input; r input; anom output; e output; a output
function [anom,e,a] = fcn(raan,inc,v,r)
    
    rnorm = abs(norm(r));
    vnorm = abs(norm(v));

    h = cross(r,v);
    hnorm = abs(norm(h));
    
    muLuna = 4.9028e12;
    
    p = (hnorm.^2)./muLuna;
    
    a = muLuna./(2.*muLuna./rnorm - vnorm.^2);
    
    e = sqrt(1 - p./a);
    
    ascnode = [cos(raan),sin(raan),0]; %Ascending node
    
    if abs(inc) > 1e-8
        if r(3) > 1e-5
            anom = acos((ascnode*r')./rnorm);
        else
            anom = 2.*pi - acos((ascnode*r')./rnorm);
        end    
    else
        if r(2) >= 0
            anom = acos((ascnode*r')./rnorm);
        else
            anom = 2.*pi - acos((ascnode*r')./rnorm);
        end 
    end
    

    
end

== matlab function SimuOrbital/Cambio ejes propulsion/MATLAB Function ==
  data: inc input; raan input; anom input; fsc input; feq output; ang input
function feq = fcn(inc,raan,anom,fsc,ang)

Reqop = [1,0,0;0,cos(inc),sin(inc);0,-sin(inc),cos(inc)]*[cos(raan),sin(raan),0;-sin(raan),cos(raan),0;0,0,1];
Ropeq = inv(Reqop);

Roplo = [1,0,0;0,0,-1;0,1,0]*[0,1,0;-1,0,0;0,0,1]*[cos(anom),sin(anom),0;-sin(anom),cos(anom),0;0,0,1];
Rloop = inv(Roplo);

alphax = ang(1);
alphay = ang(2);
alphaz = ang(3);
Rloa = [1,0,0;0,cos(alphax),sin(alphax);0,-sin(alphax),cos(alphax)]*[cos(alphay),0,-sin(alphay);0,1,0;sin(alphay),0,cos(alphay)]*[cos(alphaz),sin(alphaz),0;-sin(alphaz),cos(alphaz),0;0,0,1];
Ralo = inv(Rloa);

feq = Ropeq*Rloop*Ralo*fsc;



end
